simulink model "Ident_Motor"  (R2015a)
settings: Solver=ode23t  StartTime=0.0  StopTime=74.1  RelTol=1e-3
model workspace (MAT data in the model file):
  tpbe6446ad_f14d_43ee_8c6c_74ef65e04d1d = Simulink.SimulationData.Signal
  tpbe6446ad_f14d_43ee_8c6c_74ef65e04d1d.PortType = 'outport'
  tpbe6446ad_f14d_43ee_8c6c_74ef65e04d1d.BlockPath = Simulink.SimulationData.BlockPath
  tpbe6446ad_f14d_43ee_8c6c_74ef65e04d1d.BlockPath.path = {'Ident_Motor/In1'}
  tpbe6446ad_f14d_43ee_8c6c_74ef65e04d1d.Values = timeseries
  tpbe6446ad_f14d_43ee_8c6c_74ef65e04d1d.Values.Name = 'In1'
  tpbe6446ad_f14d_43ee_8c6c_74ef65e04d1d.Values.DataInfo = tsdata.datametadata
  tpbe6446ad_f14d_43ee_8c6c_74ef65e04d1d.Values.DataInfo.Interpolation = tsdata.interpolation
  tpbe6446ad_f14d_43ee_8c6c_74ef65e04d1d.Values.DataInfo.Interpolation.Fhandle : function handle (value not decoded)
  tpbe6446ad_f14d_43ee_8c6c_74ef65e04d1d.Values.DataInfo.Interpolation.Name = 'linear'
  tpbe6446ad_f14d_43ee_8c6c_74ef65e04d1d.Values.TimeInfo = tsdata.timemetadata
  tpbe6446ad_f14d_43ee_8c6c_74ef65e04d1d.Values.TimeInfo.Length = 1236
  tpbe6446ad_f14d_43ee_8c6c_74ef65e04d1d.Values.TimeInfo.DuplicateTimes = 0
  tpbe6446ad_f14d_43ee_8c6c_74ef65e04d1d.Values.TimeInfo.Time_ = [0 0.06 0.12 0.18 0.24 0.3 0.36 0.42 0.48 0.54 0.6 0.66 ... (1236 elements, 1236x1)]
  tpbe6446ad_f14d_43ee_8c6c_74ef65e04d1d.Values.TimeInfo.Initialized = 1
  tpbe6446ad_f14d_43ee_8c6c_74ef65e04d1d.Values.QualityInfo = tsdata.qualmetadata
  tpbe6446ad_f14d_43ee_8c6c_74ef65e04d1d.Values.Data_ = [0 0 0 0 0 0 0 0 0 0 0 0 ... (1236 elements, 1236x1)]
  tpbe6446ad_f14d_43ee_8c6c_74ef65e04d1d.Name = 'In1'
undefined symbols (not defined in the file or in its folder): b_r, J_r, Km_r, La_r
settings Model: Creator=Juan_David  LastModifiedBy=Juan_David
settings DataIOCC: ExternalInput=tpbe6446ad_f14d_43ee_8c6c_74ef65e04d1d(1)  LoadExternalInput=on  ReturnWorkspaceOutputs=on  SignalLoggingName=SDO_logsout  OutputOption=SpecifiedOutputTimes  OutputTimes=[0;0.06;0.12;0.18;0.24;0.3;0.36;0.42;0.48;0.54;0.6;0.66;0.72;0.78;0.84;0.9;0.96;1.02;1.08;1.14;1.2;1.26;1.32;1.38;1.44;1.5;1.56;1.62;1.68;1.74;1.8;1.86;1.92;1.98;2.04;2.1;2.16;2.22;2.28;2.34;2.4;2.46;2.52;2.58;2.64;2.7;2.76;2.82;2.88;2.94;3;3.06;3.12;3.18;3.24;3.3;3.36;3.42;3.48;3.54;3.6;3.66;3.72;3.78;3.84;3.9;3.96;4.02;4.08;4.14;4.2;4.26;4.32;4.38;4.44;4.5;4.56;4.62;4.68;4.74;4.8;4.86;4.92;4.98;5.04;5.1;5.16;5.22;5.28;5.34;5.4;5.46;5.52;5.58;5.64;5.7;5.76;5.82;5.88;5.94;6;6.06;6.12;6.18;6.24;6.3;6.36;6.42;6.48;6.54;6.6;6.66;6.72;6.78;6.84;6.9;6.96;7.02;7.08;7.14;7.2;7.26;7.32;7.38;7.44;7.5;7.56;7.62;7.68;7.74;7.8;7.86;7.92;7.98;8.04;8.1;8.16;8.22;8.28;8.34;8.4;8.46;8.52;8.58;8.64;8.7;8.76;8.82;8.88;8.94;9;9.06;9.12;9.18;9.24;9.3;9.36;9.42;9.48;9.54;9.6;9.66;9.72;9.78;9.84;9.9;9.96;10.02;10.08;10.14;10.2;10.26;10.32;10.38;10.44;10.5;10.56;10.62;10.68;10.74;10.8;10.86;10.92;10.98;11.04;11.1;11.16;11.22;11.28;11.34;11.4;11.46;11.52;11.58;11.64;11.7;11.76;11.82;11.88;11.94;12;12.06;12.12;12.18;12.24;12.3;12.36;12.42;12.48;12.54;12.6;12.66;12.72;12.78;12.84;12.9;12.96;13.02;13.08;13.14;13.2;13.26;13.32;13.38;13.44;13.5;13.56;13.62;13.68;13.74;13.8;13.86;13.92;13.98;14.04;14.1;14.16;14.22;14.28;14.34;14.4;14.46;14.52;14.58;14.64;14.7;14.76;14.82;14.88;14.94;15;15.06;15.12;15.18;15.24;15.3;15.36;15.42;15.48;15.54;15.6;15.66;15.72;15.78;15.84;15.9;15.96;16.02;16.08;16.14;16.2;16.26;16.32;16.38;16.44;16.5;16.56;16.62;16.68;16.74;16.8;16.86;16.92;16.98;17.04;17.1;17.16;17.22;17.28;17.34;17.4;17.46;17.52;17.58;17.64;17.7;17.76;17.82;17.88;17.94;18;18.06;18.12;18.18;18.24;18.3;18.36;18.42;18.48;18.54;18.6;18.66;18.72;18.78;18.84;18.9;18.96;19.02;19.08;19.14;19.2;19.26;19.32;19.38;19.44;19.5;19.56;19.62;19.68;19.74;19.8;19.86;19.92;19.98;20.04;20.1;20.16;20.22;20.28;20.34;20.4;20.46;20.52;20.58;20.64;20.7;20.76;20.82;20.88;20.94;21;21.06;21.12;21.18;21.24;21.3;21.36;21.42;21.48;21.54;21.6;21.66;21.72;21.78;21.84;21.9;21.96;22.02;22.08;22.14;22.2;22.26;22.32;22.38;22.44;22.5;22.56;22.62;22.68;22.74;22.8;22.86;22.92;22.98;23.04;23.1;23.16;23.22;23.28;23.34;23.4;23.46;23.52;23.58;23.64;23.7;23.76;23.82;23.88;23.94;24;24.06;24.12;24.18;24.24;24.3;24.36;24.42;24.48;24.54;24.6;24.66;24.72;24.78;24.84;24.9;24.96;25.02;25.08;25.14;25.2;25.26;25.32;25.38;25.44;25.5;25.56;25.62;25.68;25.74;25.8;25.86;25.92;25.98;26.04;26.1;26.16;26.22;26.28;26.34;26.4;26.46;26.52;26.58;26.64;26.7;26.76;26.82;26.88;26.94;27;27.06;27.12;27.18;27.24;27.3;27.36;27.42;27.48;27.54;27.6;27.66;27.72;27.78;27.84;27.9;27.96;28.02;28.08;28.14;28.2;28.26;28.32;28.38;28.44;28.5;28.56;28.62;28.68;28.74;28.8;28.86;28.92;28.98;29.04;29.1;29.16;29.22;29.28;29.34;29.4;29.46;29.52;29.58;29.64;29.7;29.76;29.82;29.88;29.94;30;30.06;30.12;30.18;30.24;30.3;30.36;30.42;30.48;30.54;30.6;30.66;30.72;30.78;30.84;30.9;30.96;31.02;31.08;31.14;31.2;31.26;31.32;31.38;31.44;31.5;31.56;31.62;31.68;31.74;31.8;31.86;31.92;31.98;32.04;32.1;32.16;32.22;32.28;32.34;32.4;32.46;32.52;32.58;32.64;32.7;32.76;32.82;32.88;32.94;33;33.06;33.12;33.18;33.24;33.3;33.36;33.42;33.48;33.54;33.6;33.66;33.72;33.78;33.84;33.9;33.96;34.02;34.08;34.14;34.2;34.26;34.32;34.38;34.44;34.5;34.56;34.62;34.68;34.74;34.8;34.86;34.92;34.98;35.04;35.1;35.16;35.22;35.28;35.34;35.4;35.46;35.52;35.58;35.64;35.7;35.76;35.82;35.88;35.94;36;36.06;36.12;36.18;36.24;36.3;36.36;36.42;36.48;36.54;36.6;36.66;36.72;36.78;36.84;36.9;36.96;37.02;37.08;37.14;37.2;37.26;37.32;37.38;37.44;37.5;37.56;37.62;37.68;37.74;37.8;37.86;37.92;37.98;38.04;38.1;38.16;38.22;38.28;38.34;38.4;38.46;38.52;38.58;38.64;38.7;38.76;38.82;38.88;38.94;39;39.06;39.12;39.18;39.24;39.3;39.36;39.42;39.48;39.54;39.6;39.66;39.72;39.78;39.84;39.9;39.96;40.02;40.08;40.14;40.2;40.26;40.32;40.38;40.44;40.5;40.56;40.62;40.68;40.74;40.8;40.86;40.92;40.98;41.04;41.1;41.16;41.22;41.28;41.34;41.4;41.46;41.52;41.58;41.64;41.7;41.76;41.82;41.88;41.94;42;42.06;42.12;42.18;42.24;42.3;42.36;42.42;42.48;42.54;42.6;42.66;42.72;42.78;42.84;42.9;42.96;43.02;43.08;43.14;43.2;43.26;43.32 ...(+2955 chars)]

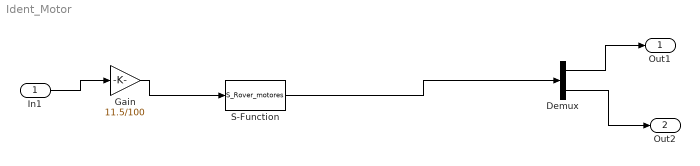
== system Ident_Motor ==
  In1 : Inport
  Demux : Demux  Outputs=2
  Gain : Gain  Gain=11.5/100
  S-Function : S-Function  FunctionName=S_Rover_motores  Parameters=Km_r,J_r,La_r,b_r
  Out1 : Outport
  Out2 : Outport  Port=2
  wires:
  Demux/1 -> Out1/1
  Demux/2 -> Out2/1
  S-Function/1 -> Demux/1
  Gain/1 -> S-Function/1
  In1/1 -> Gain/1
